simulink model "pendule_inv_echant_etu"  (R2019a)
settings: Solver=VariableStepAuto  StartTime=0.0  StopTime=10.0  RelTol=1e-3
values from neighbouring files (symbols this model uses):
  delta_t = 0.4    [simu_pendule_inv_echant_etu.m]
  g = 9.81    [simu_pendule_inv_capteur_etu.m]    (also in simu_pendule_inv_echant_etu.m; simu_pendule_inv_etu.m)
  K = [10 1]    [simu_pendule_inv_capteur_etu.m]    (also in simu_pendule_inv_echant_etu.m = [30 10]; simu_pendule_inv_etu.m = [30 10])
  l = 10    [simu_pendule_inv_capteur_etu.m]    (also in simu_pendule_inv_echant_etu.m; simu_pendule_inv_etu.m)
  ue = 0    [simu_pendule_inv_capteur_etu.m]    (also in simu_pendule_inv_echant_etu.m; simu_pendule_inv_etu.m)
  x0 = [pi/20 0]'    [simu_pendule_inv_capteur_etu.m]    (also in simu_pendule_inv_echant_etu.m; simu_pendule_inv_etu.m = [pi/10 0]')
  xe = [0 0]'    [simu_pendule_inv_capteur_etu.m]    (also in simu_pendule_inv_echant_etu.m; simu_pendule_inv_etu.m)
undefined symbols (not defined in the file or in its folder): DiscIntNeverNeededParam
settings Model: Creator=clotfi  LastModifiedBy=hmoudden

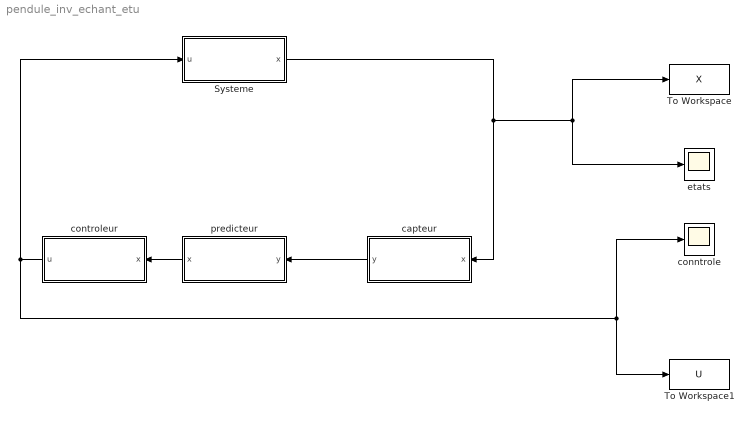
== system pendule_inv_echant_etu ==
  "Systeme " : Subsystem
  To Workspace : ToWorkspace  VariableName=X  SaveFormat=Timeseries  SampleTime=-1
  To Workspace1 : ToWorkspace  VariableName=U  SaveFormat=Timeseries  SampleTime=-1
  capteur : Subsystem
  conntrole : Scope
  controleur : Subsystem
  etats : Scope
  predicteur : Subsystem
  wires:
  controleur/1(u) -> "Systeme "/1(u), conntrole/1, To Workspace1/1
  capteur/1(y) -> predicteur/1(y)
  "Systeme "/1(x) -> To Workspace/1, etats/1, capteur/1(x)
  predicteur/1(x) -> controleur/1(x)

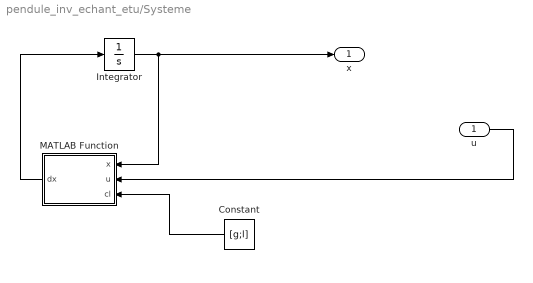
== system pendule_inv_echant_etu/Systeme  ==
  u : Inport
  Constant : Constant  Value=[g;l]
  Integrator : Integrator  InitialCondition=x0
  MATLAB Function : MATLAB Function  TreatAsAtomicUnit=on
  x : Outport
  wires:
  u/1 -> MATLAB Function/2(u)
  Constant/1 -> MATLAB Function/3(cl)
  MATLAB Function/1(dx) -> Integrator/1
  Integrator/1 -> x/1, MATLAB Function/1(x)

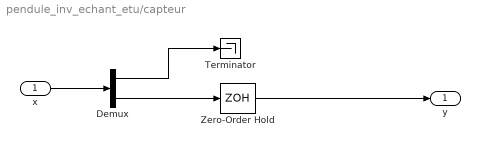
== system pendule_inv_echant_etu/capteur ==
  x : Inport
  Demux : Demux  Outputs=2
  Terminator : Terminator
  Zero-Order Hold : ZeroOrderHold  SampleTime=delta_t
  y : Outport
  wires:
  x/1 -> Demux/1
  Demux/2 -> Zero-Order Hold/1
  Demux/1 -> Terminator/1
  Zero-Order Hold/1 -> y/1

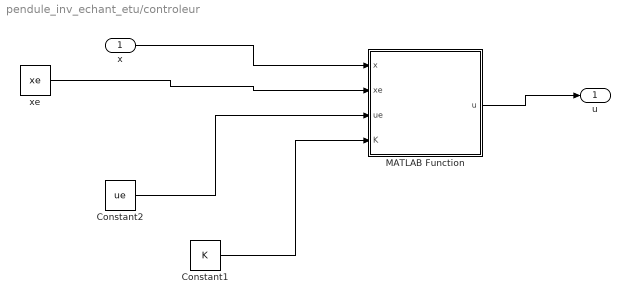
== system pendule_inv_echant_etu/controleur ==
  x : Inport
  Constant1 : Constant  Value=K
  Constant2 : Constant  Value=ue
  MATLAB Function : MATLAB Function  TreatAsAtomicUnit=on
  xe : Constant  Value=xe
  u : Outport
  wires:
  x/1 -> MATLAB Function/1(x)
  xe/1 -> MATLAB Function/2(xe)
  Constant1/1 -> MATLAB Function/4(K)
  Constant2/1 -> MATLAB Function/3(ue)
  MATLAB Function/1(u) -> u/1

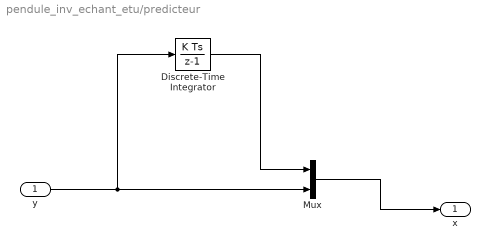
== system pendule_inv_echant_etu/predicteur ==
  y : Inport
  Discrete-Time Integrator : DiscreteIntegrator  InitialCondition=x0(1)  SampleTime=-1  ICPrevOutput=DiscIntNeverNeededParam  ICPrevScaledInput=DiscIntNeverNeededParam
  Mux : Mux  Inputs=2
  x : Outport
  wires:
  Mux/1 -> x/1
  y/1 -> Discrete-Time Integrator/1, Mux/2
  Discrete-Time Integrator/1 -> Mux/1

== matlab function pendule_inv_echant_etu/Systeme /MATLAB Function ==
  data: x input; u input; dx output; cl input
function dx = fcn(x,u,cl)
l=cl(2) ; g=cl(1);
dx=[x(2);g/l*sin(x(1))-cos(x(1))*u/l];
end

== matlab function pendule_inv_echant_etu/controleur/MATLAB Function ==
  data: x input; u output; xe input; ue input; K input
function u = fcn(x,xe,ue,K)
 u = ue+ K(:)'*( x(:)-xe(:));
end
